simulink model "simulink_app"  (R2015a)
settings: Solver=ode2  SolverMode=SingleTasking  StartTime=0.0  StopTime=inf  FixedStep=T_ctrl  RelTol=1e-3
undefined symbols (not defined in the file): A_l_max_x, A_l_max_y, A_z_max, B_hover_4dof, CG_0, epsilon, eta_23, g, h, h_M, Hover_eta_23, Hover_throtle_1, Hover_throtle_23, I_BAC_0, Ix, Iy, Iz, l, l_arm, m, m_0, m_M, Rotation_sign, T_ctrl, throtle_1, throtle_23, v_i0
libraries: XXCopter_Control x52, simulink x11, XXCopter x1
(part 4 of 4)

== matlab function simulink_app/flight_mode_effector/flight_mode_effector ==
  data: flight_mode input size=1; pos_xy_act output boolean size=1; alt_act output boolean size=1; vel_yaw_xy_act output boolean size=1; vel_yaw_z_act output boolean size=1; att_act output boolean size=1; omega_b_act output boolean size=1; pos_xy_init output size=[2,1]; alt_init output size=1; vel_yaw_xy_init output size=[2,1]; vel_yaw_z_init output size=1; att_init output size=[3,1]; b_rates_init output size=[3,1]; X_e input size=[3,1]; CA_reconf output size=1; V_yaw input size=[3,1]; Euler input size=[3,1]; omega_b input size=[3,1]; Armed output size=1
function [pos_xy_act,alt_act,vel_yaw_xy_act,vel_yaw_z_act,att_act,omega_b_act,pos_xy_init,alt_init,vel_yaw_xy_init,vel_yaw_z_init,att_init,b_rates_init,CA_reconf,Armed]   =  flight_mode_effector(flight_mode,X_e,V_yaw,Euler, omega_b)
%% Efector de los modos de vuelos
% Hace efectivos los cambios en los modos de vuelo en el controlador

%% CA_reconf
% CA_reconf = 1 : Control in 9dof with Incremental CA
% CA_reconf = 2 :  Control in 4dof with NO Incremental CA. Assumed to be a "safe" mode

%% Armed
% Armed = 0 No armed
% Armed = 1 Armed

%% Activate vectors
% 0 means no activated
% 1 means activated


switch flight_mode
    case 0 % Off
        pos_xy_act      = false;     
        alt_act         = false;
        vel_yaw_xy_act  = false; 
        vel_yaw_z_act   = false; 
        att_act         = false;
        omega_b_act     = false;
        
        pos_xy_init     = [0;0];     
        alt_init        = 0;
        vel_yaw_xy_init = [0;0]; 
        vel_yaw_z_init  = 0;
        att_init        = [0;0;0]; 
        b_rates_init    = [0;0;0];
        
        CA_reconf = 2;
        
        Armed = 0;
    case 1 % Ready
        pos_xy_act      = false;     
        alt_act         = false;
        vel_yaw_xy_act  = false; 
        vel_yaw_z_act   = false; 
        att_act         = false; 
        omega_b_act     = false;
        
        pos_xy_init     = [0;0];     
        alt_init        = 0;
        vel_yaw_xy_init = [0;0]; 
        vel_yaw_z_init  = 0;
        att_init        = [0;0;0]; 
        b_rates_init    = [0;0;0];
        
        CA_reconf = 2;
        
        Armed = 0;
    case 2 % Take off
        pos_xy_act      = true;     
        alt_act         = true;
        vel_yaw_xy_act  = true; 
        vel_yaw_z_act   = true; 
        att_act         = true; 
        omega_b_act     = true;
        
        pos_xy_init     = [0;0];    
        alt_init        = X_e(3);     
        vel_yaw_xy_init = [0;0]; 
        vel_yaw_z_init  = 0;
        att_init        = [0;0;Euler(3)]; 
        b_rates_init    = [0;0;0];
        
        CA_reconf = 1;
        
        Armed = 1;
    case 3 % Full_auto
        pos_xy_act      = true;     
        alt_act         = true;
        vel_yaw_xy_act  = true; 
        vel_yaw_z_act   = true; 
        att_act         = true; 
        omega_b_act     = true;
        
        pos_xy_init     = X_e(1:2);    
        alt_init        = X_e(3);     
        vel_yaw_xy_init = [V_yaw(1);V_yaw(2)]; 
        vel_yaw_z_init  = V_yaw(3);
        att_init        = [Euler(1);Euler(2);Euler(3)]; 
        b_rates_init    = omega_b;
        
        CA_reconf = 1;
        
        Armed = 1;
    case 4 % Vel_height_auto
        pos_xy_act      = false;     
        alt_act         = true;
        vel_yaw_xy_act  = true; 
        vel_yaw_z_act   = true; 
        att_act         = true; 
        omega_b_act     = true;
        
        pos_xy_init     = [0;0];    
        alt_init        = X_e(3);      
        vel_yaw_xy_init = [V_yaw(1);V_yaw(2)]; 
        vel_yaw_z_init  = V_yaw(3);
        att_init        = [Euler(1);Euler(2);Euler(3)]; 
        b_rates_init    = omega_b;
        
        CA_reconf = 1;
        
        Armed = 1;
    case 5 % Vel_auto
        pos_xy_act      = false;     
        alt_act         = false;
        vel_yaw_xy_act  = true; 
        vel_yaw_z_act   = true; 
        att_act         = true; 
        omega_b_act     = true;
        
        pos_xy_init     = [0;0];    
        alt_init        = 0;      
        vel_yaw_xy_init = [V_yaw(1);V_yaw(2)]; 
        vel_yaw_z_init  = V_yaw(3);
        att_init        = [Euler(1);Euler(2);Euler(3)]; 
        b_rates_init    = omega_b;
        
        CA_reconf = 1;
        
        Armed = 1;
    case 6 % Stab
        pos_xy_act      = false;     
        alt_act         = false;
        vel_yaw_xy_act  = false; 
        vel_yaw_z_act   = true; 
        att_act         = true; 
        omega_b_act     = true;
        
        pos_xy_init     = [0;0];    
        alt_init        = 0;     
        vel_yaw_xy_init = [0;0]; 
        vel_yaw_z_init  = 0;
        att_init        = [Euler(1);Euler(2);Euler(3)]; 
        b_rates_init    = omega_b;
        
        CA_reconf = 2;
        
        Armed = 1;
    case 7 % Man_ctrl
        pos_xy_act      = false;     
        alt_act         = false;
        vel_yaw_xy_act  = false; 
        vel_yaw_z_act   = true; 
        att_act         = false; 
        omega_b_act     = true;
        
        pos_xy_init     = [0;0];    
        alt_init        = 0;      
        vel_yaw_xy_init = [0;0]; 
        vel_yaw_z_init  = 0;
        att_init        = [0;0;0]; 
        b_rates_init    = [0;0;0]; 
        
        CA_reconf = 2;
        
        Armed = 1;
    case 8 % Home
        pos_xy_act      = true;     
        alt_act         = true;
        vel_yaw_xy_act  = true; 
        vel_yaw_z_act   = true; 
        att_act         = true; 
        omega_b_act     = true;
        
        pos_xy_init     = X_e(1:2);    
        alt_init        = X_e(3);      
        vel_yaw_xy_init = [V_yaw(1);V_yaw(2)]; 
        vel_yaw_z_init  = V_yaw(3);
        att_init        = [Euler(1);Euler(2);Euler(3)]; 
        b_rates_init    = omega_b; 
        
        CA_reconf = 1;
        
        Armed = 1;
        
    case 9 % Land
        pos_xy_act      = true;     
        alt_act         = true;
        vel_yaw_xy_act  = true; 
        vel_yaw_z_act   = true; 
        att_act         = true; 
        omega_b_act     = true;
        
        pos_xy_init     = X_e(1:2);    
        alt_init        = X_e(3);      
        vel_yaw_xy_init = [V_yaw(1);V_yaw(2)];
        vel_yaw_z_init  = V_yaw(3);
        att_init        = [Euler(1);Euler(2);Euler(3)]; 
        b_rates_init    = omega_b;
        
        CA_reconf = 1;
        
        Armed = 1;
    otherwise
        pos_xy_act      = false;     
        alt_act         = false;
        vel_yaw_xy_act  = false; 
        vel_yaw_z_act   = false; 
        att_act         = false; 
        omega_b_act     = false;
        
        pos_xy_init     = [0;0];    
        alt_init        = 0;      
        vel_yaw_xy_init = [0;0]; 
        vel_yaw_z_init  = 0;
        att_init        = [0;0;0]; 
        b_rates_init    = [0;0;0]; 
        
        CA_reconf = 2;
        
        Armed = 0;
        
end
